simulink subsystem "InversePendulum"  (R2023a)
settings: Solver=VariableStepAuto  StartTime=0.0  StopTime=10.0  RelTol=1e-3
model mask{M_p=0.2, m_st=0.1, l=1, g=9.81}
settings Model: Creator=Лиза  LastModifiedBy=user

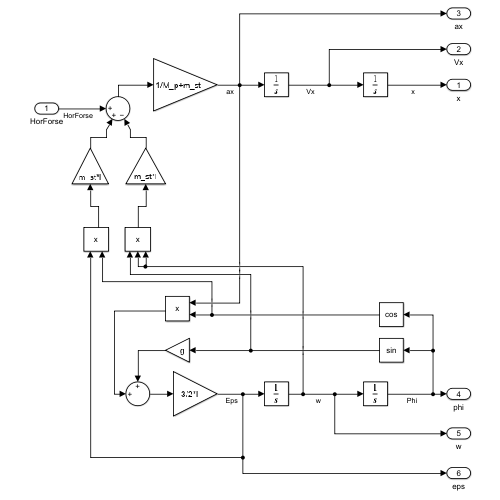
[thumbnail: Simulink's stored preview of the top-level diagram]
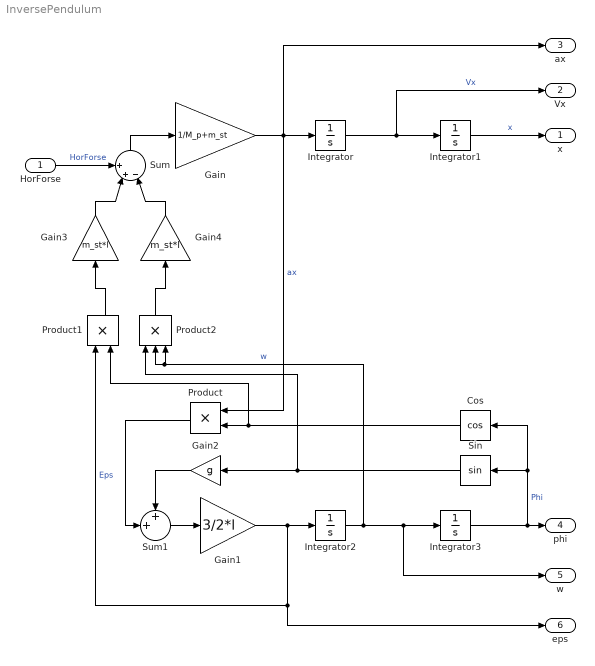
== system InversePendulum ==
  HorForse : Inport
  Cos : Trigonometry  Operator=cos
  Gain : Gain  Gain=1/M_p+m_st
  Gain1 : Gain  Gain=3/2*l
  Gain2 : Gain  Gain=g
  Gain3 : Gain  Gain=m_st*l
  Gain4 : Gain  Gain=m_st*l
  Integrator : Integrator
  Integrator1 : Integrator
  Integrator2 : Integrator
  Integrator3 : Integrator  InitialCondition=5
  Product : Product
  Product1 : Product
  Product2 : Product  Inputs=3
  Sin : Trigonometry
  Sum : Sum  Inputs=++-|
  Sum1 : Sum  Inputs=++|
  x : Outport
  Vx : Outport  Port=2
  ax : Outport  Port=3
  phi : Outport  Port=4
  w : Outport  Port=5
  eps : Outport  Port=6
  wires:
  Gain/1 -> ax/1, Integrator/1, Product/1  "ax"
  Integrator/1 -> Vx/1, Integrator1/1  "Vx"
  Sum1/1 -> Gain1/1
  Integrator2/1 -> Product2/3, Product2/2, w/1, Integrator3/1  "w"
  Integrator1/1 -> x/1  "x"
  Integrator3/1 -> Cos/1, Sin/1, phi/1  "Phi"
  HorForse/1 -> Sum/1  "HorForse"
  Sum/1 -> Gain/1
  Gain1/1 -> Product1/1, eps/1, Integrator2/1  "Eps"
  Gain2/1 -> Sum1/1
  Sin/1 -> Gain2/1, Product2/1
  Cos/1 -> Product/2, Product1/2
  Product/1 -> Sum1/2
  Product1/1 -> Gain3/1
  Gain3/1 -> Sum/2
  Gain4/1 -> Sum/3
  Product2/1 -> Gain4/1
